simulink model "csgv_simulinkmodel (2)"  (R2023a)
settings: Solver=VariableStepAuto  StartTime=0.0  StopTime=500  RelTol=1e-3
values from neighbouring files (symbols this model uses):
  Af = 2.33    [input_info (2).m]
  Cd = 0.28    [input_info (2).m]
  elev_date_1 = date_elev(:,1)    [input_info (2).m]
  elev_date_2 = date_elev(:,2)    [input_info (2).m]
  eta = 0.93    [input_info (2).m]
  fr = 0.015    [input_info (2).m]
  g = 9.81    [input_info (2).m]
  m = 1521    [input_info (2).m]
  R = 0.5    [input_info (2).m]
  rho = 1.2    [input_info (2).m]
  slope_date_1 = date_slope(:,1)    [input_info (2).m]
  slope_date_2_degree = zeros(length(slope_date_2_grad),1)    [input_info (2).m]
undefined symbols (not defined in the file or in its folder): sigbuilder_block
libraries: mpclib x1
settings Model: Creator=91807  LastModifiedBy=metha
settings ModelReferenceCC: EnableRefExpFcnMdlSchedulingChecks=on

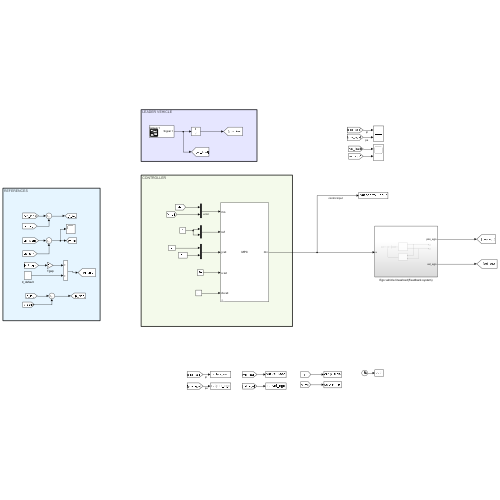
[thumbnail: Simulink's stored preview of the top-level diagram]
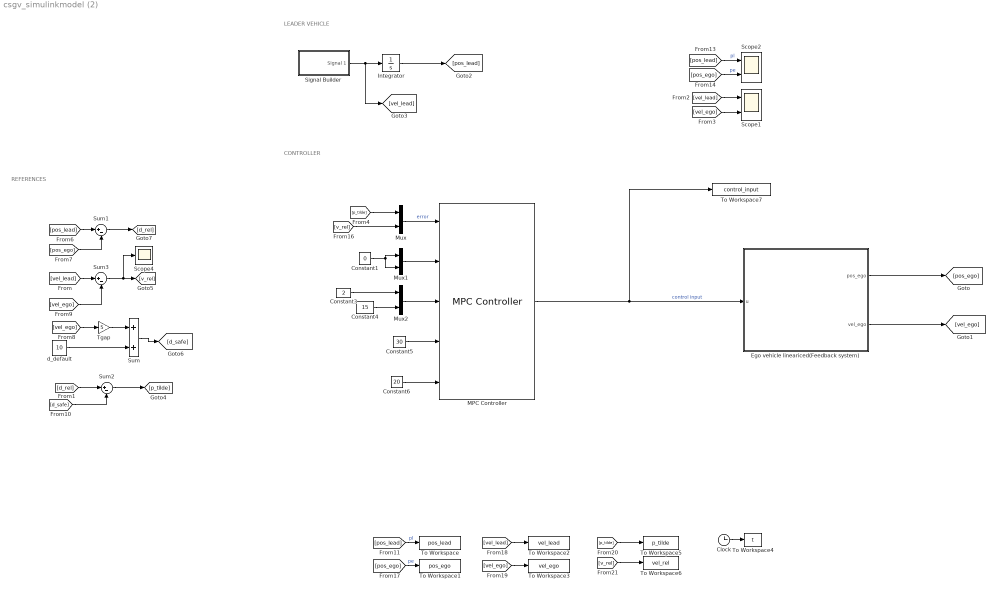
== system csgv_simulinkmodel (2) ==
  note: CONTROLLER
  note: REFERENCES
  note: LEADER VEHICLE
  Clock : Clock
  Constant1 : Constant  Value=0
  Constant3 : Constant  Value=2
  Constant4 : Constant  Value=15
  Constant5 : Constant  Value=30
  Constant6 : Constant  Value=20
  Ego vehicle lineariced(Feedback system) : Subsystem
  Integrator : Integrator
  MPC Controller : mpclib/MPC Controller  SCDEnableBlockLinearizationSpecification=on  mpcobj=mpc1  is_multiple=0  enable_value=0  return_u0=off  updateMPCinCallerWorkspace=on  md_inport=off  mv_inport=off  uref_inport=off  return_cost=off  return_mvseq=off  return_qpstatus=off  return_xseq=off  return_state=off  return_ovseq=off  state_inport=off  umin_inport=off  umax_inport=off  ymin_inport=off  ymax_inport=off  cc_inport=off  ywt_inport=on  uwt_inport=on  duwt_inport=on  rhoeps_inport=off  pm_inport=off  MaximumP=10  HorizonChoice=FixedHorizon  n_ts=0.1  n_p=50  n_mv=1  n_md=0  n_ud=0  n_mo=2  n_uo=0  BlockDataType=double  SampleTimeInherited=off  switch_inport=off
  Mux : Mux  Inputs=2
  Mux1 : Mux  Inputs=2
  Mux2 : Mux  Inputs=2
  Scope1 : Scope  NumInputPorts=2
  Scope2 : Scope  NumInputPorts=2
  Scope4 : Scope
  Signal Builder : Subsystem  Tag=STV Subsys  LoadFcn=sigbuilder_block('load');  StartFcn=sigbuilder_block('start');  StopFcn=sigbuilder_block('stop');  ClipboardFcn=sigbuilder_block('clipboard');  mask(Sigbuilder block){tuvar=[0:10]}
      mask help: Simulink:masks:SigbuilderBlock_MD
      mask init:
      | if ~strcmp(get_param(bdroot(gcbh),'SimulationStatus'),'stopped') tuvar = sigbuilder_block('maskInit'); end
      settings: CopyFcn=sigbuilder_block('copy');  DeleteFcn=sigbuilder_block('delete');  ModelCloseFcn=sigbuilder_block('modelClose');  PreSaveFcn=sigbuilder_block('preSave');  PauseFcn=sigbuilder_block('pause');  ContinueFcn=sigbuilder_block('continue');  NameChangeFcn=sigbuilder_block('namechange');  OpenFcn=sigbuilder_block('open',[438 182.4 550.8 400.2 ]);  CloseFcn=sigbuilder_block('close');
      mask Display: plot(0, 0, 100, 100,[2, 2, 32, 32, 2], [68, 8, 8, 68, 68],[32, 2], [38, 38], [32, 19, 2],[53, 60, 44], [32, 17, 17, 2],[16, 16, 31, 31]);txt = getActiveGroup(gcbh);text(2, 100, txt,'verticalAlignment', 'top');
  Sum : Sum
  Sum1 : Sum  Inputs=|+-
  Sum2 : Sum  Inputs=|+-
  Sum3 : Sum  Inputs=|+-
  Tgap : Gain  Gain=5
  To Workspace : ToWorkspace  VariableName=pos_lead  SampleTime=-1
      settings: Save2DSignal=2-D array (concatenate along first dimension)
  To Workspace1 : ToWorkspace  VariableName=pos_ego  SampleTime=-1
      settings: Save2DSignal=2-D array (concatenate along first dimension)
  To Workspace2 : ToWorkspace  VariableName=vel_lead  SampleTime=-1
      settings: Save2DSignal=2-D array (concatenate along first dimension)
  To Workspace3 : ToWorkspace  VariableName=vel_ego  SampleTime=-1
      settings: Save2DSignal=2-D array (concatenate along first dimension)
  To Workspace4 : ToWorkspace  VariableName=t  SampleTime=-1
      settings: Save2DSignal=2-D array (concatenate along first dimension)
  To Workspace5 : ToWorkspace  VariableName=p_tilde  SampleTime=-1
      settings: Save2DSignal=2-D array (concatenate along first dimension)
  To Workspace6 : ToWorkspace  VariableName=vel_rel  SampleTime=-1
      settings: Save2DSignal=2-D array (concatenate along first dimension)
  To Workspace7 : ToWorkspace  VariableName=control_input  SampleTime=-1
      settings: Save2DSignal=2-D array (concatenate along first dimension)
  d_default : Constant  Value=10
  wires:
  Ego vehicle lineariced(Feedback system)/1(pos_ego) -> [pos_ego]
  Ego vehicle lineariced(Feedback system)/2(vel_ego) -> [vel_ego]
  Clock/1 -> To Workspace4/1
  [vel_lead] -> To Workspace2/1
  [pos_ego] -> To Workspace1/1  "pe"
  [pos_lead] -> To Workspace/1  "pl"
  [v_rel] -> To Workspace6/1
  [vel_ego] -> To Workspace3/1
  [p_tilde] -> To Workspace5/1
  Signal Builder/1(Signal 1) -> [vel_lead], Integrator/1
  Integrator/1 -> [pos_lead]
  [vel_ego] -> Scope1/2
  [vel_lead] -> Scope1/1
  [pos_ego] -> Scope2/2  "pe"
  [pos_lead] -> Scope2/1  "pl"
  [pos_ego] -> Sum1/2
  Sum1/1 -> [d_rel]
  [vel_ego] -> Sum3/2
  [d_rel] -> Sum2/1
  [d_safe] -> Sum2/2
  Sum/1 -> [d_safe]
  d_default/1 -> Sum/2
  Sum3/1 -> Scope4/1, [v_rel]
  [vel_ego] -> Tgap/1
  [vel_lead] -> Sum3/1
  [pos_lead] -> Sum1/1
  Tgap/1 -> Sum/1
  Sum2/1 -> [p_tilde]
  MPC Controller/1 -> To Workspace7/1, Ego vehicle lineariced(Feedback system)/1(u)  "control input"
  Constant4/1 -> Mux2/2
  [v_rel] -> Mux/2
  Mux1/1 -> MPC Controller/2
  [p_tilde] -> Mux/1
  Constant1/1 -> Mux1/1, Mux1/2
  Constant3/1 -> Mux2/1
  Mux/1 -> MPC Controller/1  "error"
  Constant6/1 -> MPC Controller/5
  Constant5/1 -> MPC Controller/4
  Mux2/1 -> MPC Controller/3

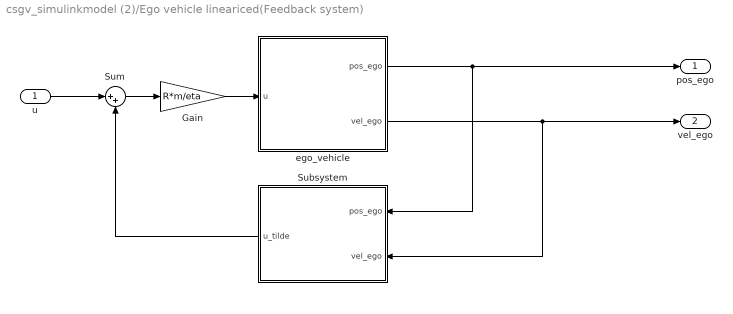
== system csgv_simulinkmodel (2)/Ego vehicle lineariced(Feedback system) ==
  u : Inport
  Gain : Gain  Gain=R*m/eta
  Subsystem : Subsystem
  Sum : Sum  Inputs=|++
  ego_vehicle : Subsystem
  pos_ego : Outport
  vel_ego : Outport  Port=2
  wires:
  Gain/1 -> ego_vehicle/1(u)
  ego_vehicle/2(vel_ego) -> vel_ego/1, Subsystem/2(vel_ego)
  ego_vehicle/1(pos_ego) -> pos_ego/1, Subsystem/1(pos_ego)
  Subsystem/1(u_tilde) -> Sum/2
  u/1 -> Sum/1
  Sum/1 -> Gain/1

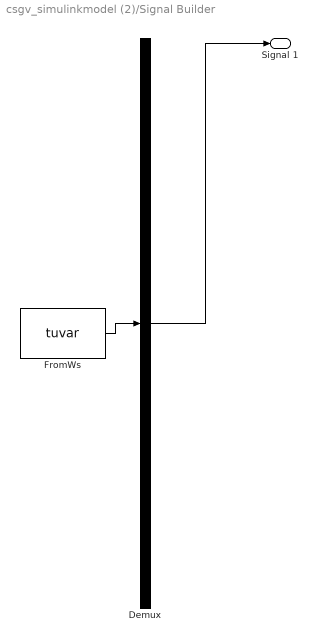
== system csgv_simulinkmodel (2)/Signal Builder ==
  Demux : Demux  Tag=STV Demux  Outputs=1
      settings: DisplayOption=none
  FromWs : FromWorkspace  Tag=STV FromWs  VariableName=tuvar
      SigBuilderData=|
      | common.afterFinalStr = 'Extrapolate'
      | common.sampleTime = 0
      | dataSet.timeRange = [0 400]
      | dataSet.name = 'Group 1'
      | sbobj.Groups.Name = 'Group 1'
      | sbobj.Groups.Signals.Name = 'Signal 1'
      | sbobj.Groups.Signals.XData = [0 75 75 150 150 200 200 275 275 350 350 400]
      | sbobj.Groups.Signals.YData = [18 18 10 10 20 20 15 15 5 5 0 0]
      | sbobj.Groups.TimeRange = [0 400]
  Signal 1 : Outport  Tag=STV Outport
  wires:
  Demux/1 -> Signal 1/1
  FromWs/1 -> Demux/1

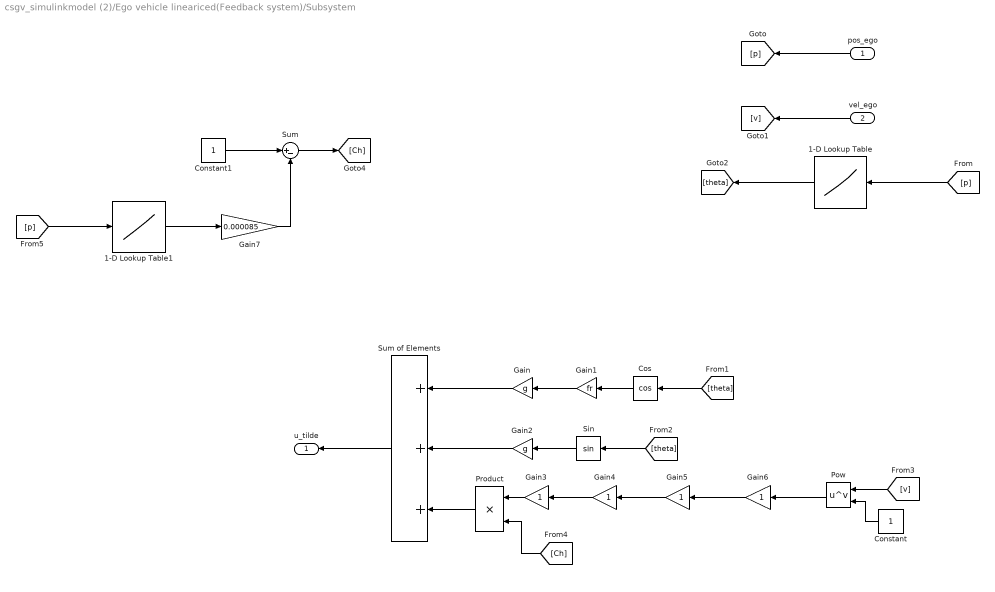
== system csgv_simulinkmodel (2)/Ego vehicle lineariced(Feedback system)/Subsystem ==
  pos_ego : Inport
  vel_ego : Inport  Port=2
  1-D Lookup Table : Lookup_n-D  NumberOfTableDimensions=1  BreakpointsForDimension1=slope_date_1  Table=slope_date_2_degree  InternalRulePriority=Speed  RndMeth=Simplest
  1-D Lookup Table1 : Lookup_n-D  NumberOfTableDimensions=1  BreakpointsForDimension1=elev_date_1  Table=elev_date_2  InternalRulePriority=Speed  RndMeth=Simplest
  Constant : Constant
  Constant1 : Constant
  Cos : Trigonometry  Operator=cos
  Gain : Gain  Gain=g
  Gain1 : Gain  Gain=fr
  Gain2 : Gain  Gain=g
  Gain{3..6} (4 alike) : Gain
  Gain7 : Gain  Gain=0.000085
  Pow : Math  Operator=pow  SignedPower=on  RndMeth=Zero
  Product : Product
  Sin : Trigonometry
  Sum : Sum  Inputs=|+-
  Sum of Elements : Sum  Inputs=+++
  u_tilde : Outport
  wires:
  pos_ego/1 -> [p]
  vel_ego/1 -> [v]
  Gain/1 -> Sum of Elements/1
  Gain1/1 -> Gain/1
  Gain2/1 -> Sum of Elements/2
  Cos/1 -> Gain1/1
  Sin/1 -> Gain2/1
  [theta] -> Cos/1
  [theta] -> Sin/1
  Product/1 -> Sum of Elements/3
  Gain3/1 -> Product/1
  Gain4/1 -> Gain3/1
  Gain5/1 -> Gain4/1
  Gain6/1 -> Gain5/1
  Pow/1 -> Gain6/1
  [v] -> Pow/1
  Constant/1 -> Pow/2
  [Ch] -> Product/2
  Sum of Elements/1 -> u_tilde/1
  1-D Lookup Table1/1 -> Gain7/1
  [p] -> 1-D Lookup Table1/1
  Gain7/1 -> Sum/2
  Sum/1 -> [Ch]
  Constant1/1 -> Sum/1
  [p] -> 1-D Lookup Table/1
  1-D Lookup Table/1 -> [theta]

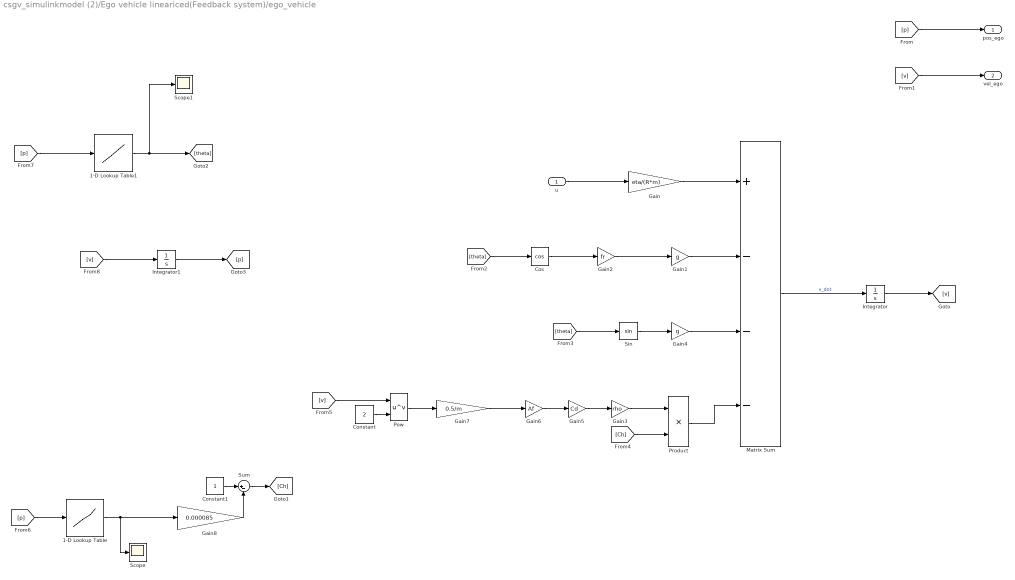
== system csgv_simulinkmodel (2)/Ego vehicle lineariced(Feedback system)/ego_vehicle ==
  u : Inport
  1-D Lookup Table : Lookup_n-D  NumberOfTableDimensions=1  BreakpointsForDimension1=elev_date_1  Table=elev_date_2  InternalRulePriority=Speed  RndMeth=Simplest
  1-D Lookup Table1 : Lookup_n-D  NumberOfTableDimensions=1  BreakpointsForDimension1=slope_date_1  Table=slope_date_2_degree  InternalRulePriority=Speed  RndMeth=Simplest
  Constant : Constant  Value=2
  Constant1 : Constant
  Cos : Trigonometry  Operator=cos
  Gain : Gain  Gain=eta/(R*m)
  Gain1 : Gain  Gain=g
  Gain2 : Gain  Gain=fr
  Gain3 : Gain  Gain=rho
  Gain4 : Gain  Gain=g
  Gain5 : Gain  Gain=Cd
  Gain6 : Gain  Gain=Af
  Gain7 : Gain  Gain=0.5/m
  Gain8 : Gain  Gain=0.000085
  Integrator : Integrator
  Integrator1 : Integrator
  Matrix Sum : Sum  Inputs=+---
  Pow : Math  Operator=pow  SignedPower=on  RndMeth=Zero
  Product : Product
  Scope : Scope
  Scope1 : Scope
  Sin : Trigonometry
  Sum : Sum  Inputs=|+-
  pos_ego : Outport
  vel_ego : Outport  Port=2
  wires:
  u/1 -> Gain/1
  1-D Lookup Table1/1 -> Scope1/1, [theta]
  [v] -> Integrator1/1
  [v] -> vel_ego/1
  Integrator/1 -> [v]
  Gain1/1 -> Matrix Sum/2
  Pow/1 -> Gain7/1
  1-D Lookup Table/1 -> Scope/1, Gain8/1
  [p] -> pos_ego/1
  [p] -> 1-D Lookup Table1/1
  Gain5/1 -> Gain3/1
  Sin/1 -> Gain4/1
  Product/1 -> Matrix Sum/4
  Gain/1 -> Matrix Sum/1
  Gain3/1 -> Product/1
  Gain8/1 -> Sum/2
  [theta] -> Sin/1
  Constant1/1 -> Sum/1
  [theta] -> Cos/1
  Gain7/1 -> Gain6/1
  [p] -> 1-D Lookup Table/1
  [Ch] -> Product/2
  [v] -> Pow/1
  Matrix Sum/1 -> Integrator/1  "v_dot"
  Cos/1 -> Gain2/1
  Constant/1 -> Pow/2
  Gain6/1 -> Gain5/1
  Sum/1 -> [Ch]
  Gain2/1 -> Gain1/1
  Gain4/1 -> Matrix Sum/3
  Integrator1/1 -> [p]
